simulink model "ACC_Scenario_006_cs"  (R2014b)
settings: Solver=ode5  SolverMode=SingleTasking  StartTime=0.0  StopTime=inf  FixedStep=1/100  RelTol=1e-3
PreLoadFcn:
  | mbxruntime.callbacks.PreLoadFcn(bdroot);
  | check_NUTS_defined;
  | 
  | assignin('base',['model_closed_' bdroot],false);addpath('../includes_ACC');
PostLoadFcn:
  | mbxruntime.callbacks.PostLoadFcn(bdroot);
InitFcn:
  | mbxruntime.callbacks.InitFcn(bdroot);
StartFcn:
  | mbxruntime.callbacks.StartFcn(bdroot);
StopFcn:
  | mbxruntime.callbacks.StopFcn(bdroot);
model workspace: external: MAT-File .\ACC_Scenario_006_cs_hws.mat (data not in the file)
undefined symbols (not defined in the file or in its folder): mbxruntime, OrientationPitch, OrientationRoll, PositionX, PositionY, PositionZ, tabledata, warningInitialVelocity, x0
undefined symbols (not defined in the file): ACC_Scenario_006_cs_061450488d6753c4, ACC_Scenario_006_cs_13896134c615b72a, ACC_Scenario_006_cs_18eaf2a52f2ef75d, ACC_Scenario_006_cs_59e375456829d2f0, ACC_Scenario_006_cs_8a2109b915871f11, ACC_Scenario_006_cs_a4f79cab717c06e2, ACC_Scenario_006_cs_Audi_A8_1_Dynamics_Simple_initialPitch, ACC_Scenario_006_cs_Audi_A8_1_Dynamics_Simple_initialRoll, ACC_Scenario_006_cs_Audi_A8_1_Dynamics_Simple_initialX, ACC_Scenario_006_cs_Audi_A8_1_Dynamics_Simple_initialY, ACC_Scenario_006_cs_Audi_A8_1_Dynamics_Simple_initialYaw, ACC_Scenario_006_cs_Audi_A8_1_Dynamics_Simple_initialZ, ACC_Scenario_006_cs_BMW_X5_1_Path_pathUniqueID, ACC_Scenario_006_cs_BMW_X5_1_SpeedProfile_speedProfileUniqueID, ACC_Scenario_006_cs_e4633c18fd34a832, ACC_Scenario_006_cs_f83c81dc10cd364a, ACC_Scenario_006_cs_Fiat_Bravo_1_Path_pathUniqueID, ACC_Scenario_006_cs_Ford_Fiesta_1_Path_pathUniqueID, ACC_Scenario_006_cs_Honda_Pan_European_1_Path_pathUniqueID, ACC_Scenario_006_cs_Mazda_RX8_1_Path_pathUniqueID, ACC_Scenario_006_cs_Sphere_1_Dynamics_Empty_STATE_Sphere_1_x0, ACC_Scenario_006_cs_Sphere_1_Dynamics_Empty_STATE_Sphere_1_y0, ACC_Scenario_006_cs_Sphere_1_Dynamics_Empty_STATE_Sphere_1_Yaw0, ACC_Scenario_006_cs_Sphere_1_Dynamics_Empty_STATE_Sphere_1_z0, ACC_Scenario_006_cs_Toyota_Yaris_1_Path_pathUniqueID, SteeringColumn, SteeringWheel, Wheel0, Wheel0_Suspension, Wheel1, Wheel1_Suspension, WheelL0, WheelL1, WheelR0, WheelR1
libraries: simulink_extras x60, simulink x21, PreScanSimulinkLibrary x5, PreScanUsefulBlocks x2
(part 9 of 24)

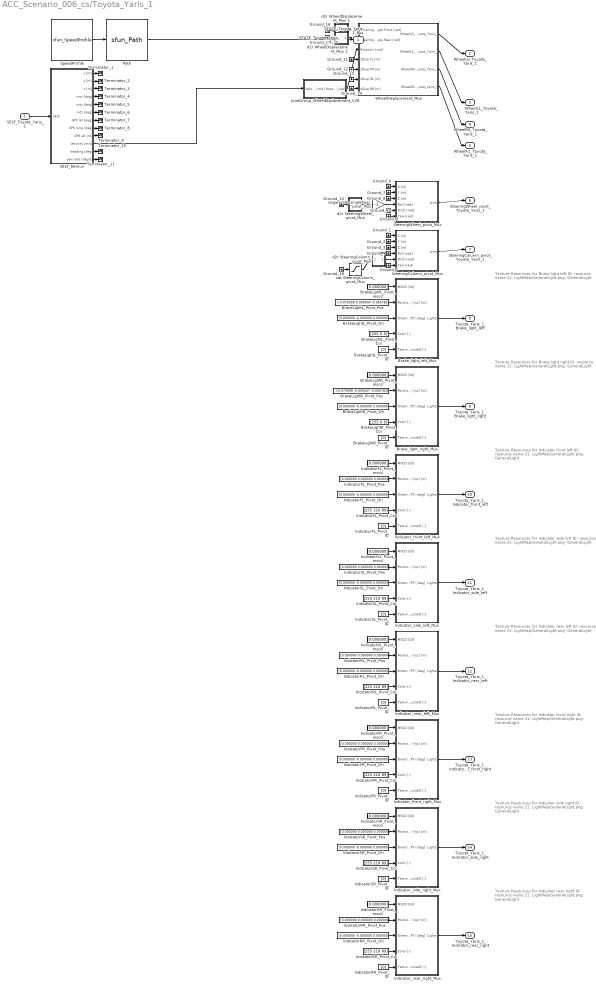
== system ACC_Scenario_006_cs/Toyota_Yaris_1 ==
  note: Texture Resources for Brake light left
      |
      | ID: resource name
      | 21: LightMap\GeneralLight.png: GeneralLight
  note: Texture Resources for Brake light right
      |
      | ID: resource name
      | 21: LightMap\GeneralLight.png: GeneralLight
  note: Texture Resources for Indicator front left
      |
      | ID: resource name
      | 21: LightMap\GeneralLight.png: GeneralLight
  note: Texture Resources for Indicator side left
      |
      | ID: resource name
      | 21: LightMap\GeneralLight.png: GeneralLight
  note: Texture Resources for Indicator rear left
      |
      | ID: resource name
      | 21: LightMap\GeneralLight.png: GeneralLight
  note: Texture Resources for Indicator front right
      |
      | ID: resource name
      | 21: LightMap\GeneralLight.png: GeneralLight
  note: Texture Resources for Indicator side right
      |
      | ID: resource name
      | 21: LightMap\GeneralLight.png: GeneralLight
  note: Texture Resources for Indicator rear right
      |
      | ID: resource name
      | 21: LightMap\GeneralLight.png: GeneralLight
  SELF_Toyota_Yaris_1 : Inport  Tag=inport/SelfPort  OutDataTypeStr=Bus: PRESCAN_SELFSENSORDATA  PortDimensions=1  SampleTime=1/100  BusOutputAsStruct=on
  BrakeLightL_Pivot_Col : Constant  Tag=VisuLightConst  Value=[255 0 0]
  BrakeLightL_Pivot_ID : Constant  Tag=VisuLightConst  Value=[0]
  BrakeLightL_Pivot_Ori : Constant  Tag=VisuLightConst  Value=[0.000000 -0.000000 0.000000]
  BrakeLightL_Pivot_Pos : Constant  Tag=VisuLightConst  Value=[-0.073098 0.009000 -0.060782]
  BrakeLightL_Pivot_mscd : Constant  Tag=VisuLightConst  Value=[0.000000]
  BrakeLightR_Pivot_Col : Constant  Tag=VisuLightConst  Value=[255 0 0]
  BrakeLightR_Pivot_ID : Constant  Tag=VisuLightConst  Value=[0]
  BrakeLightR_Pivot_Ori : Constant  Tag=VisuLightConst  Value=[0.000000 -0.000000 0.000000]
  BrakeLightR_Pivot_Pos : Constant  Tag=VisuLightConst  Value=[-0.073098 -0.009447 -0.060782]
  BrakeLightR_Pivot_mscd : Constant  Tag=VisuLightConst  Value=[0.000000]
  Brake_light_left_Mux : Subsystem  Tag=mux/ActiveLight  mask(PreScan User Interface: VisuActiveLight){}
      mask help:
      | The VisuActiveLight block provides a way for detailed animation of Light Sources, such as the indicator, brake, fog and main lights of a vehicle, or a light post.
      |
      | For more information, please click Help.
      settings: DeleteFcn=PreScanBlockDeleteFcn;
      mask Help: eval('openHelp(209)')
  Brake_light_right_Mux : Subsystem  Tag=mux/ActiveLight  mask(PreScan User Interface: VisuActiveLight){}
      mask help:
      | The VisuActiveLight block provides a way for detailed animation of Light Sources, such as the indicator, brake, fog and main lights of a vehicle, or a light post.
      |
      | For more information, please click Help.
      settings: DeleteFcn=PreScanBlockDeleteFcn;
      mask Help: eval('openHelp(209)')
  Ground_{1..18} (18 alike) : Ground
  IndicatorFL_Pivot_Col : Constant  Tag=VisuLightConst  Value=[255 210 89]
  IndicatorFL_Pivot_ID : Constant  Tag=VisuLightConst  Value=[0]
  IndicatorFL_Pivot_Ori : Constant  Tag=VisuLightConst  Value=[0.000000 -0.000000 0.000000]
  IndicatorFL_Pivot_Pos : Constant  Tag=VisuLightConst  Value=[0.000000 0.000000 0.000000]
  IndicatorFL_Pivot_mscd : Constant  Tag=VisuLightConst  Value=[0.000000]
  IndicatorFR_Pivot_Col : Constant  Tag=VisuLightConst  Value=[255 210 89]
  IndicatorFR_Pivot_ID : Constant  Tag=VisuLightConst  Value=[0]
  IndicatorFR_Pivot_Ori : Constant  Tag=VisuLightConst  Value=[0.000000 -0.000000 0.000000]
  IndicatorFR_Pivot_Pos : Constant  Tag=VisuLightConst  Value=[0.000000 0.000000 0.000000]
  IndicatorFR_Pivot_mscd : Constant  Tag=VisuLightConst  Value=[0.000000]
  IndicatorRL_Pivot_Col : Constant  Tag=VisuLightConst  Value=[255 210 89]
  IndicatorRL_Pivot_ID : Constant  Tag=VisuLightConst  Value=[0]
  IndicatorRL_Pivot_Ori : Constant  Tag=VisuLightConst  Value=[0.000000 -0.000000 0.000000]
  IndicatorRL_Pivot_Pos : Constant  Tag=VisuLightConst  Value=[0.000000 0.000000 0.000000]
  IndicatorRL_Pivot_mscd : Constant  Tag=VisuLightConst  Value=[0.000000]
  IndicatorRR_Pivot_Col : Constant  Tag=VisuLightConst  Value=[255 210 89]
  IndicatorRR_Pivot_ID : Constant  Tag=VisuLightConst  Value=[0]
  IndicatorRR_Pivot_Ori : Constant  Tag=VisuLightConst  Value=[0.000000 -0.000000 0.000000]
  IndicatorRR_Pivot_Pos : Constant  Tag=VisuLightConst  Value=[0.000000 0.000000 0.000000]
  IndicatorRR_Pivot_mscd : Constant  Tag=VisuLightConst  Value=[0.000000]
  IndicatorSL_Pivot_Col : Constant  Tag=VisuLightConst  Value=[255 210 89]
  IndicatorSL_Pivot_ID : Constant  Tag=VisuLightConst  Value=[0]
  IndicatorSL_Pivot_Ori : Constant  Tag=VisuLightConst  Value=[0.000000 -0.000000 0.000000]
  IndicatorSL_Pivot_Pos : Constant  Tag=VisuLightConst  Value=[0.000000 0.000000 0.000000]
  IndicatorSL_Pivot_mscd : Constant  Tag=VisuLightConst  Value=[0.000000]
  IndicatorSR_Pivot_Col : Constant  Tag=VisuLightConst  Value=[255 210 89]
  IndicatorSR_Pivot_ID : Constant  Tag=VisuLightConst  Value=[0]
  IndicatorSR_Pivot_Ori : Constant  Tag=VisuLightConst  Value=[0.000000 -0.000000 0.000000]
  IndicatorSR_Pivot_Pos : Constant  Tag=VisuLightConst  Value=[0.000000 0.000000 0.000000]
  IndicatorSR_Pivot_mscd : Constant  Tag=VisuLightConst  Value=[0.000000]
  Indicator_front_left_Mux : Subsystem  Tag=mux/ActiveLight  mask(PreScan User Interface: VisuActiveLight){}
      mask help:
      | The VisuActiveLight block provides a way for detailed animation of Light Sources, such as the indicator, brake, fog and main lights of a vehicle, or a light post.
      |
      | For more information, please click Help.
      settings: DeleteFcn=PreScanBlockDeleteFcn;
      mask Help: eval('openHelp(209)')
  Indicator_front_right_Mux : Subsystem  Tag=mux/ActiveLight  mask(PreScan User Interface: VisuActiveLight){}
      mask help:
      | The VisuActiveLight block provides a way for detailed animation of Light Sources, such as the indicator, brake, fog and main lights of a vehicle, or a light post.
      |
      | For more information, please click Help.
      settings: DeleteFcn=PreScanBlockDeleteFcn;
      mask Help: eval('openHelp(209)')
  Indicator_rear_left_Mux : Subsystem  Tag=mux/ActiveLight  mask(PreScan User Interface: VisuActiveLight){}
      mask help:
      | The VisuActiveLight block provides a way for detailed animation of Light Sources, such as the indicator, brake, fog and main lights of a vehicle, or a light post.
      |
      | For more information, please click Help.
      settings: DeleteFcn=PreScanBlockDeleteFcn;
      mask Help: eval('openHelp(209)')
  Indicator_rear_right_Mux : Subsystem  Tag=mux/ActiveLight  mask(PreScan User Interface: VisuActiveLight){}
      mask help:
      | The VisuActiveLight block provides a way for detailed animation of Light Sources, such as the indicator, brake, fog and main lights of a vehicle, or a light post.
      |
      | For more information, please click Help.
      settings: DeleteFcn=PreScanBlockDeleteFcn;
      mask Help: eval('openHelp(209)')
  Indicator_side_left_Mux : Subsystem  Tag=mux/ActiveLight  mask(PreScan User Interface: VisuActiveLight){}
      mask help:
      | The VisuActiveLight block provides a way for detailed animation of Light Sources, such as the indicator, brake, fog and main lights of a vehicle, or a light post.
      |
      | For more information, please click Help.
      settings: DeleteFcn=PreScanBlockDeleteFcn;
      mask Help: eval('openHelp(209)')
  Indicator_side_right_Mux : Subsystem  Tag=mux/ActiveLight  mask(PreScan User Interface: VisuActiveLight){}
      mask help:
      | The VisuActiveLight block provides a way for detailed animation of Light Sources, such as the indicator, brake, fog and main lights of a vehicle, or a light post.
      |
      | For more information, please click Help.
      settings: DeleteFcn=PreScanBlockDeleteFcn;
      mask Help: eval('openHelp(209)')
  JointGroup_WheelDisplacement_V2R : Subsystem  Tag=mux/Wheels  mask(PreScan Velocity to Wheel Angle Block:){TimeStep=1/100, TireRadius=0.29}
      mask prompts: TimeStep "Auto Assigned: Time Step [s]"; TireRadius "Tire Radius [m]"
      settings: DeleteFcn=PreScanBlockDeleteFcn;
      mask Display: disp('Velocity\nto\nWheelAngle')
  Path : S-Function  Tag=Path  LoadFcn=load('PrescanMotionData.mat')  FunctionName=sfun_Path  Parameters=uniqueID, pathUniqueID, timestep  EnableBusSupport=off  mask(Path){uniqueID=359, pathUniqueID=ACC_Scenario_006_cs_Toyota_Yaris_1_Path_pathUniqueID, timestep=1/100}
      mask prompts: uniqueID "Object Unique ID"; pathUniqueID "Path Unique ID"; timestep "MATLAB timestep:"
      mask help:
      | The path block outputs the position along a given trajectory.
      |
      | For more information, please click Help.
      mask Help: eval('openHelp(312)')
      mask Display: image(imread('Path.png'))
  SELF_Demux : Subsystem  Tag=demux/SelfPort  mask(PreScan Demux Block:){}
      mask help:
      | The SELF port shows (state) information of the actor itself. The outputs are position in the experiment's axis system and the GPS coordinates, and the object's absolute velocity and compass heading.
      |
      | For more information, please click Help.
      settings: DeleteFcn=PreScanBlockDeleteFcn;
      mask Help: eval('openHelp(462)')
      mask Display:
      | port_label('output',1,'x [m]')
      | port_label('output',2,'y [m]')
      | port_label('output',3,'z [m]','texmode','on')
      | port_label('output',4,'Rotx [deg]','texmode','on')
      | port_label('output',5,'Roty [deg]','texmode','on')
      | port_label('output',6,'Rotz [deg]','texmode','on')
      | port_label('output',7,'GPS lat [deg]','texmode','on')
      | port_label('output',8,'GPS long [deg]','texmode','on')
      | port_label('output',9,'GPS alt [m]','texmode','on')
      | port_label('output',10,'Velocity [m/s]')
      | port_label('output',11,'Heading [deg]')
      | port_label('output',12,'Yaw rate [deg/s]')
  STATE_Toyota_Yaris_1_rc : RateTransition  Tag=mux_rc/StatePort  OutPortSampleTimeOpt=Inherit
  SpeedProfile : S-Function  Tag=SpeedProfile  LoadFcn=load('PrescanMotionData.mat')  FunctionName=sfun_SpeedProfile  Parameters=speedProfileUniqueID, timestep  EnableBusSupport=off  mask(SpeedProfile){speedProfileUniqueID=ACC_Scenario_006_cs_13896134c615b72a, timestep=1/100}
      mask prompts: speedProfileUniqueID "Speed Profile Unique ID"; timestep "MATLAB timestep:"
      mask help:
      | The speed profile block outputs the travelled distance, velocities and acceleration along a given path.
      |
      | For more information, please click Help.
      mask Help: eval('openHelp(312)')
      mask Display: image(imread('SpeedProfile.png'))
  SteeringColumn_pivot_Mux : Subsystem  Tag=mux/Joint  mask(PreScan Mux Block){DisplayName=SteeringColumn}
      mask prompts: DisplayName "Display Name"
      mask help:
      | This block simulates a generic joint used for generic models. This joint can be enabled/disabled from the GUI.
      |
      | For more information, please click Help.
      settings: DeleteFcn=PreScanBlockDeleteFcn;
      mask Help: eval('openHelp(254)')
  SteeringWheel_pivot_Mux : Subsystem  Tag=mux/Joint  mask(PreScan Mux Block){DisplayName=SteeringWheel}
      mask prompts: DisplayName "Display Name"
      mask help:
      | This block simulates a generic joint used for generic models. This joint can be enabled/disabled from the GUI.
      |
      | For more information, please click Help.
      settings: DeleteFcn=PreScanBlockDeleteFcn;
      mask Help: eval('openHelp(254)')
  Terminator_{1..11} (11 alike) : Terminator
  WheelDisplacement_Mux : Subsystem  Tag=mux/JointGroup  mask(JointGroup){}
      mask help:
      | The JointGroup allows to control several Joints in one go, as defined for this particular model.
      | For more information, look in the PreScan manual in the section "Model Preparation Tool" -> "Joint Groups"
      |
      | For more information on the Joints simulink interface, press Help.
      mask Help: eval('openHelp(254)')
  d2r SteeringColumn_pivot_Mux : Subsystem  mask(DegreesToRadians){}
      mask help: SimulinkBlocks:simulink_extras:DegreesToRadians_MD
      mask Help: web([docroot '/simulink/ref_extras/degreestoradians.html'])
      mask Display: disp('D2R')
  d2r SteeringWheel_pivot_Mux : Subsystem  mask(DegreesToRadians){}
      mask help: SimulinkBlocks:simulink_extras:DegreesToRadians_MD
      mask Help: web([docroot '/simulink/ref_extras/degreestoradians.html'])
      mask Display: disp('D2R')
  d2r WheelDisplacement_Mux 1 : Subsystem  mask(DegreesToRadians){}
      mask help: SimulinkBlocks:simulink_extras:DegreesToRadians_MD
      mask Help: web([docroot '/simulink/ref_extras/degreestoradians.html'])
      mask Display: disp('D2R')
  d2r WheelDisplacement_Mux 2 : Subsystem  mask(DegreesToRadians){}
      mask help: SimulinkBlocks:simulink_extras:DegreesToRadians_MD
      mask Help: web([docroot '/simulink/ref_extras/degreestoradians.html'])
      mask Display: disp('D2R')
  negate SteeringWheel_pivot_Mux : Gain  Gain=-1
  sat SteeringColumn_pivot_Mux : Saturate  UpperLimit=30  LowerLimit=-5
  STATE_Toyota_Yaris_1_bus : Outport  Tag=outport/StatePort  OutDataTypeStr=Bus: PRESCAN_STATEACTUATORDATA  PortDimensions=1  SampleTime=1/100
  WheelL0_Toyota_Yaris_1 : Outport  Tag=outport/JointActuator  Port=2  OutDataTypeStr=Bus: PRESCAN_POSE_DATA  SampleTime=1/100
  WheelL1_Toyota_Yaris_1 : Outport  Tag=outport/JointActuator  Port=3  OutDataTypeStr=Bus: PRESCAN_POSE_DATA  SampleTime=1/100
  WheelR0_Toyota_Yaris_1 : Outport  Tag=outport/JointActuator  Port=4  OutDataTypeStr=Bus: PRESCAN_POSE_DATA  SampleTime=1/100
  WheelR1_Toyota_Yaris_1 : Outport  Tag=outport/JointActuator  Port=5  OutDataTypeStr=Bus: PRESCAN_POSE_DATA  SampleTime=1/100
  SteeringWheel_pivot_Toyota_Yaris_1 : Outport  Tag=outport/JointActuator  Port=6  OutDataTypeStr=Bus: PRESCAN_POSE_DATA  SampleTime=1/100
  SteeringColumn_pivot_Toyota_Yaris_1 : Outport  Tag=outport/JointActuator  Port=7  OutDataTypeStr=Bus: PRESCAN_POSE_DATA  SampleTime=1/100
  Toyota_Yaris_1_Brake_light_left : Outport  Tag=outport/BrakeLightL_Pivot  Port=8  OutDataTypeStr=Bus: PRESCAN_VISULIGHTACTUATOR_DATA  SampleTime=1/100
  Toyota_Yaris_1_Brake_light_right : Outport  Tag=outport/BrakeLightR_Pivot  Port=9  OutDataTypeStr=Bus: PRESCAN_VISULIGHTACTUATOR_DATA  SampleTime=1/100
  Toyota_Yaris_1_Indicator_front_left : Outport  Tag=outport/IndicatorFL_Pivot  Port=10  OutDataTypeStr=Bus: PRESCAN_VISULIGHTACTUATOR_DATA  SampleTime=1/100
  Toyota_Yaris_1_Indicator_side_left : Outport  Tag=outport/IndicatorSL_Pivot  Port=11  OutDataTypeStr=Bus: PRESCAN_VISULIGHTACTUATOR_DATA  SampleTime=1/100
  Toyota_Yaris_1_Indicator_rear_left : Outport  Tag=outport/IndicatorRL_Pivot  Port=12  OutDataTypeStr=Bus: PRESCAN_VISULIGHTACTUATOR_DATA  SampleTime=1/100
  Toyota_Yaris_1_Indicator_front_right : Outport  Tag=outport/IndicatorFR_Pivot  Port=13  OutDataTypeStr=Bus: PRESCAN_VISULIGHTACTUATOR_DATA  SampleTime=1/100
  Toyota_Yaris_1_Indicator_side_right : Outport  Tag=outport/IndicatorSR_Pivot  Port=14  OutDataTypeStr=Bus: PRESCAN_VISULIGHTACTUATOR_DATA  SampleTime=1/100
  Toyota_Yaris_1_Indicator_rear_right : Outport  Tag=outport/IndicatorRR_Pivot  Port=15  OutDataTypeStr=Bus: PRESCAN_VISULIGHTACTUATOR_DATA  SampleTime=1/100
  wires:
  sat SteeringColumn_pivot_Mux/1 -> d2r SteeringColumn_pivot_Mux/1(Degrees in)
  d2r SteeringColumn_pivot_Mux/1(Radians out) -> SteeringColumn_pivot_Mux/5(Pitch [rad])
  d2r SteeringWheel_pivot_Mux/1(Radians out) -> negate SteeringWheel_pivot_Mux/1
  negate SteeringWheel_pivot_Mux/1 -> SteeringWheel_pivot_Mux/4(Roll [rad])
  d2r WheelDisplacement_Mux 1/1(Radians out) -> WheelDisplacement_Mux/1(Steering Angle Front [rad])
  d2r WheelDisplacement_Mux 2/1(Radians out) -> WheelDisplacement_Mux/2(Steering Angle Rear [rad])
  SELF_Demux/10(velocity [m/s]) -> JointGroup_WheelDisplacement_V2R/1(Velocity [m/s])
  STATE_Toyota_Yaris_1_rc/1 -> STATE_Toyota_Yaris_1_bus/1
  SpeedProfile/1 -> Path/1
  Path/1 -> STATE_Toyota_Yaris_1_rc/1
  SELF_Toyota_Yaris_1/1 -> SELF_Demux/1(SELF)
  WheelDisplacement_Mux/1(WheelL0_Toyota_Yaris_1) -> WheelL0_Toyota_Yaris_1/1
  WheelDisplacement_Mux/2(WheelL1_Toyota_Yaris_1) -> WheelL1_Toyota_Yaris_1/1
  WheelDisplacement_Mux/3(WheelR0_Toyota_Yaris_1) -> WheelR0_Toyota_Yaris_1/1
  WheelDisplacement_Mux/4(WheelR1_Toyota_Yaris_1) -> WheelR1_Toyota_Yaris_1/1
  JointGroup_WheelDisplacement_V2R/1(Rotation [rad]) -> WheelDisplacement_Mux/3(Rotation [rad])
  SteeringWheel_pivot_Mux/1(Joint) -> SteeringWheel_pivot_Toyota_Yaris_1/1
  SteeringColumn_pivot_Mux/1(Joint) -> SteeringColumn_pivot_Toyota_Yaris_1/1
  Brake_light_left_Mux/1(Lights) -> Toyota_Yaris_1_Brake_light_left/1
  BrakeLightL_Pivot_mscd/1 -> Brake_light_left_Mux/1(MSCD [Cd])
  BrakeLightL_Pivot_Pos/1 -> Brake_light_left_Mux/2(Position (xyz) [m])
  BrakeLightL_Pivot_Ori/1 -> Brake_light_left_Mux/3(Orientation (RPY) [deg])
  BrakeLightL_Pivot_Col/1 -> Brake_light_left_Mux/4(Color [-])
  BrakeLightL_Pivot_ID/1 -> Brake_light_left_Mux/5(TextureResourceID [-])
  Brake_light_right_Mux/1(Lights) -> Toyota_Yaris_1_Brake_light_right/1
  BrakeLightR_Pivot_mscd/1 -> Brake_light_right_Mux/1(MSCD [Cd])
  BrakeLightR_Pivot_Pos/1 -> Brake_light_right_Mux/2(Position (xyz) [m])
  BrakeLightR_Pivot_Ori/1 -> Brake_light_right_Mux/3(Orientation (RPY) [deg])
  BrakeLightR_Pivot_Col/1 -> Brake_light_right_Mux/4(Color [-])
  BrakeLightR_Pivot_ID/1 -> Brake_light_right_Mux/5(TextureResourceID [-])
  Indicator_front_left_Mux/1(Lights) -> Toyota_Yaris_1_Indicator_front_left/1
  IndicatorFL_Pivot_mscd/1 -> Indicator_front_left_Mux/1(MSCD [Cd])
  IndicatorFL_Pivot_Pos/1 -> Indicator_front_left_Mux/2(Position (xyz) [m])
  IndicatorFL_Pivot_Ori/1 -> Indicator_front_left_Mux/3(Orientation (RPY) [deg])
  IndicatorFL_Pivot_Col/1 -> Indicator_front_left_Mux/4(Color [-])
  IndicatorFL_Pivot_ID/1 -> Indicator_front_left_Mux/5(TextureResourceID [-])
  Indicator_side_left_Mux/1(Lights) -> Toyota_Yaris_1_Indicator_side_left/1
  IndicatorSL_Pivot_mscd/1 -> Indicator_side_left_Mux/1(MSCD [Cd])
  IndicatorSL_Pivot_Pos/1 -> Indicator_side_left_Mux/2(Position (xyz) [m])
  IndicatorSL_Pivot_Ori/1 -> Indicator_side_left_Mux/3(Orientation (RPY) [deg])
  IndicatorSL_Pivot_Col/1 -> Indicator_side_left_Mux/4(Color [-])
  IndicatorSL_Pivot_ID/1 -> Indicator_side_left_Mux/5(TextureResourceID [-])
  Indicator_rear_left_Mux/1(Lights) -> Toyota_Yaris_1_Indicator_rear_left/1
  IndicatorRL_Pivot_mscd/1 -> Indicator_rear_left_Mux/1(MSCD [Cd])
  IndicatorRL_Pivot_Pos/1 -> Indicator_rear_left_Mux/2(Position (xyz) [m])
  IndicatorRL_Pivot_Ori/1 -> Indicator_rear_left_Mux/3(Orientation (RPY) [deg])
  IndicatorRL_Pivot_Col/1 -> Indicator_rear_left_Mux/4(Color [-])
  IndicatorRL_Pivot_ID/1 -> Indicator_rear_left_Mux/5(TextureResourceID [-])
  Indicator_front_right_Mux/1(Lights) -> Toyota_Yaris_1_Indicator_front_right/1
  IndicatorFR_Pivot_mscd/1 -> Indicator_front_right_Mux/1(MSCD [Cd])
  IndicatorFR_Pivot_Pos/1 -> Indicator_front_right_Mux/2(Position (xyz) [m])
  IndicatorFR_Pivot_Ori/1 -> Indicator_front_right_Mux/3(Orientation (RPY) [deg])
  IndicatorFR_Pivot_Col/1 -> Indicator_front_right_Mux/4(Color [-])
  IndicatorFR_Pivot_ID/1 -> Indicator_front_right_Mux/5(TextureResourceID [-])
  Indicator_side_right_Mux/1(Lights) -> Toyota_Yaris_1_Indicator_side_right/1
  IndicatorSR_Pivot_mscd/1 -> Indicator_side_right_Mux/1(MSCD [Cd])
  IndicatorSR_Pivot_Pos/1 -> Indicator_side_right_Mux/2(Position (xyz) [m])
  IndicatorSR_Pivot_Ori/1 -> Indicator_side_right_Mux/3(Orientation (RPY) [deg])
  IndicatorSR_Pivot_Col/1 -> Indicator_side_right_Mux/4(Color [-])
  IndicatorSR_Pivot_ID/1 -> Indicator_side_right_Mux/5(TextureResourceID [-])
  Indicator_rear_right_Mux/1(Lights) -> Toyota_Yaris_1_Indicator_rear_right/1
  IndicatorRR_Pivot_mscd/1 -> Indicator_rear_right_Mux/1(MSCD [Cd])
  IndicatorRR_Pivot_Pos/1 -> Indicator_rear_right_Mux/2(Position (xyz) [m])
  IndicatorRR_Pivot_Ori/1 -> Indicator_rear_right_Mux/3(Orientation (RPY) [deg])
  IndicatorRR_Pivot_Col/1 -> Indicator_rear_right_Mux/4(Color [-])
  IndicatorRR_Pivot_ID/1 -> Indicator_rear_right_Mux/5(TextureResourceID [-])
  SELF_Demux/1(x [m]) -> Terminator_1/1
  SELF_Demux/2(y [m]) -> Terminator_2/1
  SELF_Demux/3(z [m]) -> Terminator_3/1
  SELF_Demux/4(rotx [deg]) -> Terminator_4/1
  SELF_Demux/5(roty [deg]) -> Terminator_5/1
  SELF_Demux/6(rotz [deg]) -> Terminator_6/1
  SELF_Demux/7(GPS lat [deg]) -> Terminator_7/1
  SELF_Demux/8(GPS long [deg]) -> Terminator_8/1
  SELF_Demux/9(GPS alt [m]) -> Terminator_9/1
  SELF_Demux/11(heading [deg]) -> Terminator_10/1
  SELF_Demux/12(yaw rate [deg/s]) -> Terminator_11/1
  Ground_1/1 -> SteeringColumn_pivot_Mux/1(X [m])
  Ground_2/1 -> SteeringColumn_pivot_Mux/2(Y [m])
  Ground_3/1 -> SteeringColumn_pivot_Mux/3(Z [m])
  Ground_4/1 -> SteeringColumn_pivot_Mux/4(Roll [rad])
  Ground_5/1 -> SteeringColumn_pivot_Mux/6(Yaw [rad])
  Ground_6/1 -> SteeringWheel_pivot_Mux/1(X [m])
  Ground_7/1 -> SteeringWheel_pivot_Mux/2(Y [m])
  Ground_8/1 -> SteeringWheel_pivot_Mux/3(Z [m])
  Ground_9/1 -> SteeringWheel_pivot_Mux/5(Pitch [rad])
  Ground_10/1 -> SteeringWheel_pivot_Mux/6(Yaw [rad])
  Ground_11/1 -> WheelDisplacement_Mux/4(zDisp FL [m])
  Ground_12/1 -> WheelDisplacement_Mux/5(zDisp FR [m])
  Ground_13/1 -> WheelDisplacement_Mux/6(zDisp RL [m])
  Ground_14/1 -> WheelDisplacement_Mux/7(zDisp RR [m])
  Ground_15/1 -> d2r SteeringWheel_pivot_Mux/1(Degrees in)
  Ground_16/1 -> d2r WheelDisplacement_Mux 1/1(Degrees in)
  Ground_17/1 -> d2r WheelDisplacement_Mux 2/1(Degrees in)
  Ground_18/1 -> sat SteeringColumn_pivot_Mux/1

== system ACC_Scenario_006_cs/Toyota_Yaris_1_Brake_light_left ==
  Toyota_Yaris_1_Brake_light_left : Inport  Tag=inport/BrakeLightL_Pivot  OutDataTypeStr=Bus: PRESCAN_VISULIGHTACTUATOR_DATA  SampleTime=1/100  BusOutputAsStruct=on
  Actuator : S-Function  FunctionName=sfun_VisuLightActuator  Parameters=mbxruntime.parameters.convert(UniqueID), mbxruntime.parameters.convert(LightName), mbxruntime.parameters.convert(PivotName), mbxruntime.parameters.convert(TextureResources), mbxruntime.parameters.convert(ColorsObjectName), mbxruntime.parameters.convert(MeshOnColor), mbxruntime.parameters.convert(MeshOffColor),tabledata, TimeStep  EnableBusSupport=off  mask(PreScan Sink Block: VisuActiveLight){UniqueID=359, LightName=Toyota_Yaris_1.LightActuator_0_BrakeLightL_ActiveLight, PivotName=Toyota_Yaris_1.BrakeLightL_Pivot, TextureResources={ '21' 'LightMap\GeneralLight.png'}, ColorsObjectName=Toyota_Yaris_1.BrakeLightL, MeshOnColor=[255    0    0  255  255    0    0  255  102  102  102  255  510    0    0  255], MeshOffColor=[255    0    0  255  255    0    0  255  102  102  102  255    0    0    0  255], TimeStep=1/100}
      mask prompts: UniqueID "Parent Unique Identifier"; LightName "Light"; PivotName "Pivot"; TextureResources "Texture Resources"; ColorsObjectName "Light Fixture Color Object"; MeshOnColor "Light Fixture On Color"; MeshOffColor "Light Fixture Off Color"; TimeStep "Simulink time step"
      mask help:
      | The VisuActiveLight block provides a way for detailed animation of Light Sources, such as the indicator, brake, fog and main lights of a vehicle, or a light post.
      |
      | For more information, please click Help.
      mask init:
      | [tabledata] = mbxruntime.parameters.table(UniqueID,LightName,PivotName,TextureResources,ColorsObjectName,MeshOnColor,MeshOffColor);
      mask Help: eval('openHelp(209)')
      mask Display: image(imread('HeadLight.png'))
  wires:
  Toyota_Yaris_1_Brake_light_left/1 -> Actuator/1

== system ACC_Scenario_006_cs/Toyota_Yaris_1_Brake_light_right ==
  Toyota_Yaris_1_Brake_light_right : Inport  Tag=inport/BrakeLightR_Pivot  OutDataTypeStr=Bus: PRESCAN_VISULIGHTACTUATOR_DATA  SampleTime=1/100  BusOutputAsStruct=on
  Actuator : S-Function  FunctionName=sfun_VisuLightActuator  Parameters=mbxruntime.parameters.convert(UniqueID), mbxruntime.parameters.convert(LightName), mbxruntime.parameters.convert(PivotName), mbxruntime.parameters.convert(TextureResources), mbxruntime.parameters.convert(ColorsObjectName), mbxruntime.parameters.convert(MeshOnColor), mbxruntime.parameters.convert(MeshOffColor),tabledata, TimeStep  EnableBusSupport=off  mask(PreScan Sink Block: VisuActiveLight){UniqueID=359, LightName=Toyota_Yaris_1.LightActuator_1_BrakeLightR_ActiveLight, PivotName=Toyota_Yaris_1.BrakeLightR_Pivot, TextureResources={ '21' 'LightMap\GeneralLight.png'}, ColorsObjectName=Toyota_Yaris_1.BrakeLightR, MeshOnColor=[255    0    0  255  255    0    0  255  102  102  102  255  510    0    0  255], MeshOffColor=[255    0    0  255  255    0    0  255  102  102  102  255    0    0    0  255], TimeStep=1/100}
      mask prompts: UniqueID "Parent Unique Identifier"; LightName "Light"; PivotName "Pivot"; TextureResources "Texture Resources"; ColorsObjectName "Light Fixture Color Object"; MeshOnColor "Light Fixture On Color"; MeshOffColor "Light Fixture Off Color"; TimeStep "Simulink time step"
      mask help:
      | The VisuActiveLight block provides a way for detailed animation of Light Sources, such as the indicator, brake, fog and main lights of a vehicle, or a light post.
      |
      | For more information, please click Help.
      mask init:
      | [tabledata] = mbxruntime.parameters.table(UniqueID,LightName,PivotName,TextureResources,ColorsObjectName,MeshOnColor,MeshOffColor);
      mask Help: eval('openHelp(209)')
      mask Display: image(imread('HeadLight.png'))
  wires:
  Toyota_Yaris_1_Brake_light_right/1 -> Actuator/1

== system ACC_Scenario_006_cs/Toyota_Yaris_1_Indicator_front_left ==
  Toyota_Yaris_1_Indicator_front_left : Inport  Tag=inport/IndicatorFL_Pivot  OutDataTypeStr=Bus: PRESCAN_VISULIGHTACTUATOR_DATA  SampleTime=1/100  BusOutputAsStruct=on
  Actuator : S-Function  FunctionName=sfun_VisuLightActuator  Parameters=mbxruntime.parameters.convert(UniqueID), mbxruntime.parameters.convert(LightName), mbxruntime.parameters.convert(PivotName), mbxruntime.parameters.convert(TextureResources), mbxruntime.parameters.convert(ColorsObjectName), mbxruntime.parameters.convert(MeshOnColor), mbxruntime.parameters.convert(MeshOffColor),tabledata, TimeStep  EnableBusSupport=off  mask(PreScan Sink Block: VisuActiveLight){UniqueID=359, LightName=Toyota_Yaris_1.LightActuator_6_IndicatorFL_ActiveLight, PivotName=Toyota_Yaris_1.IndicatorFL_Pivot, TextureResources={ '21' 'LightMap\GeneralLight.png'}, ColorsObjectName=Toyota_Yaris_1.IndicatorFL, MeshOnColor=[255  165    0    0  255  165    0    0  102  102  102  255  510  420  178  255], MeshOffColor=[255  165    0    0  255  165    0    0  102  102  102  255    0    0    0  255], TimeStep=1/100}
      mask prompts: UniqueID "Parent Unique Identifier"; LightName "Light"; PivotName "Pivot"; TextureResources "Texture Resources"; ColorsObjectName "Light Fixture Color Object"; MeshOnColor "Light Fixture On Color"; MeshOffColor "Light Fixture Off Color"; TimeStep "Simulink time step"
      mask help:
      | The VisuActiveLight block provides a way for detailed animation of Light Sources, such as the indicator, brake, fog and main lights of a vehicle, or a light post.
      |
      | For more information, please click Help.
      mask init:
      | [tabledata] = mbxruntime.parameters.table(UniqueID,LightName,PivotName,TextureResources,ColorsObjectName,MeshOnColor,MeshOffColor);
      mask Help: eval('openHelp(209)')
      mask Display: image(imread('HeadLight.png'))
  wires:
  Toyota_Yaris_1_Indicator_front_left/1 -> Actuator/1

== system ACC_Scenario_006_cs/Toyota_Yaris_1_Indicator_front_right ==
  Toyota_Yaris_1_Indicator_front_right : Inport  Tag=inport/IndicatorFR_Pivot  OutDataTypeStr=Bus: PRESCAN_VISULIGHTACTUATOR_DATA  SampleTime=1/100  BusOutputAsStruct=on
  Actuator : S-Function  FunctionName=sfun_VisuLightActuator  Parameters=mbxruntime.parameters.convert(UniqueID), mbxruntime.parameters.convert(LightName), mbxruntime.parameters.convert(PivotName), mbxruntime.parameters.convert(TextureResources), mbxruntime.parameters.convert(ColorsObjectName), mbxruntime.parameters.convert(MeshOnColor), mbxruntime.parameters.convert(MeshOffColor),tabledata, TimeStep  EnableBusSupport=off  mask(PreScan Sink Block: VisuActiveLight){UniqueID=359, LightName=Toyota_Yaris_1.LightActuator_9_IndicatorFR_ActiveLight, PivotName=Toyota_Yaris_1.IndicatorFR_Pivot, TextureResources={ '21' 'LightMap\GeneralLight.png'}, ColorsObjectName=Toyota_Yaris_1.IndicatorFR, MeshOnColor=[255  165    0    0  255  165    0    0  102  102  102  255  510  420  178  255], MeshOffColor=[255  165    0    0  255  165    0    0  102  102  102  255    0    0    0  255], TimeStep=1/100}
      mask prompts: UniqueID "Parent Unique Identifier"; LightName "Light"; PivotName "Pivot"; TextureResources "Texture Resources"; ColorsObjectName "Light Fixture Color Object"; MeshOnColor "Light Fixture On Color"; MeshOffColor "Light Fixture Off Color"; TimeStep "Simulink time step"
      mask help:
      | The VisuActiveLight block provides a way for detailed animation of Light Sources, such as the indicator, brake, fog and main lights of a vehicle, or a light post.
      |
      | For more information, please click Help.
      mask init:
      | [tabledata] = mbxruntime.parameters.table(UniqueID,LightName,PivotName,TextureResources,ColorsObjectName,MeshOnColor,MeshOffColor);
      mask Help: eval('openHelp(209)')
      mask Display: image(imread('HeadLight.png'))
  wires:
  Toyota_Yaris_1_Indicator_front_right/1 -> Actuator/1

== system ACC_Scenario_006_cs/Toyota_Yaris_1_Indicator_rear_left ==
  Toyota_Yaris_1_Indicator_rear_left : Inport  Tag=inport/IndicatorRL_Pivot  OutDataTypeStr=Bus: PRESCAN_VISULIGHTACTUATOR_DATA  SampleTime=1/100  BusOutputAsStruct=on
  Actuator : S-Function  FunctionName=sfun_VisuLightActuator  Parameters=mbxruntime.parameters.convert(UniqueID), mbxruntime.parameters.convert(LightName), mbxruntime.parameters.convert(PivotName), mbxruntime.parameters.convert(TextureResources), mbxruntime.parameters.convert(ColorsObjectName), mbxruntime.parameters.convert(MeshOnColor), mbxruntime.parameters.convert(MeshOffColor),tabledata, TimeStep  EnableBusSupport=off  mask(PreScan Sink Block: VisuActiveLight){UniqueID=359, LightName=Toyota_Yaris_1.LightActuator_8_IndicatorRL_ActiveLight, PivotName=Toyota_Yaris_1.IndicatorRL_Pivot, TextureResources={ '21' 'LightMap\GeneralLight.png'}, ColorsObjectName=Toyota_Yaris_1.IndicatorRL, MeshOnColor=[255  165    0    0  255  165    0    0  102  102  102  255  510  420  178  255], MeshOffColor=[255  165    0    0  255  165    0    0  102  102  102  255    0    0    0  255], TimeStep=1/100}
      mask prompts: UniqueID "Parent Unique Identifier"; LightName "Light"; PivotName "Pivot"; TextureResources "Texture Resources"; ColorsObjectName "Light Fixture Color Object"; MeshOnColor "Light Fixture On Color"; MeshOffColor "Light Fixture Off Color"; TimeStep "Simulink time step"
      mask help:
      | The VisuActiveLight block provides a way for detailed animation of Light Sources, such as the indicator, brake, fog and main lights of a vehicle, or a light post.
      |
      | For more information, please click Help.
      mask init:
      | [tabledata] = mbxruntime.parameters.table(UniqueID,LightName,PivotName,TextureResources,ColorsObjectName,MeshOnColor,MeshOffColor);
      mask Help: eval('openHelp(209)')
      mask Display: image(imread('HeadLight.png'))
  wires:
  Toyota_Yaris_1_Indicator_rear_left/1 -> Actuator/1

== system ACC_Scenario_006_cs/Toyota_Yaris_1_Indicator_rear_right ==
  Toyota_Yaris_1_Indicator_rear_right : Inport  Tag=inport/IndicatorRR_Pivot  OutDataTypeStr=Bus: PRESCAN_VISULIGHTACTUATOR_DATA  SampleTime=1/100  BusOutputAsStruct=on
  Actuator : S-Function  FunctionName=sfun_VisuLightActuator  Parameters=mbxruntime.parameters.convert(UniqueID), mbxruntime.parameters.convert(LightName), mbxruntime.parameters.convert(PivotName), mbxruntime.parameters.convert(TextureResources), mbxruntime.parameters.convert(ColorsObjectName), mbxruntime.parameters.convert(MeshOnColor), mbxruntime.parameters.convert(MeshOffColor),tabledata, TimeStep  EnableBusSupport=off  mask(PreScan Sink Block: VisuActiveLight){UniqueID=359, LightName=Toyota_Yaris_1.LightActuator_11_IndicatorRR_ActiveLight, PivotName=Toyota_Yaris_1.IndicatorRR_Pivot, TextureResources={ '21' 'LightMap\GeneralLight.png'}, ColorsObjectName=Toyota_Yaris_1.IndicatorRR, MeshOnColor=[255  165    0    0  255  165    0    0  102  102  102  255  510  420  178  255], MeshOffColor=[255  165    0    0  255  165    0    0  102  102  102  255    0    0    0  255], TimeStep=1/100}
      mask prompts: UniqueID "Parent Unique Identifier"; LightName "Light"; PivotName "Pivot"; TextureResources "Texture Resources"; ColorsObjectName "Light Fixture Color Object"; MeshOnColor "Light Fixture On Color"; MeshOffColor "Light Fixture Off Color"; TimeStep "Simulink time step"
      mask help:
      | The VisuActiveLight block provides a way for detailed animation of Light Sources, such as the indicator, brake, fog and main lights of a vehicle, or a light post.
      |
      | For more information, please click Help.
      mask init:
      | [tabledata] = mbxruntime.parameters.table(UniqueID,LightName,PivotName,TextureResources,ColorsObjectName,MeshOnColor,MeshOffColor);
      mask Help: eval('openHelp(209)')
      mask Display: image(imread('HeadLight.png'))
  wires:
  Toyota_Yaris_1_Indicator_rear_right/1 -> Actuator/1

== system ACC_Scenario_006_cs/Toyota_Yaris_1_Indicator_side_left ==
  Toyota_Yaris_1_Indicator_side_left : Inport  Tag=inport/IndicatorSL_Pivot  OutDataTypeStr=Bus: PRESCAN_VISULIGHTACTUATOR_DATA  SampleTime=1/100  BusOutputAsStruct=on
  Actuator : S-Function  FunctionName=sfun_VisuLightActuator  Parameters=mbxruntime.parameters.convert(UniqueID), mbxruntime.parameters.convert(LightName), mbxruntime.parameters.convert(PivotName), mbxruntime.parameters.convert(TextureResources), mbxruntime.parameters.convert(ColorsObjectName), mbxruntime.parameters.convert(MeshOnColor), mbxruntime.parameters.convert(MeshOffColor),tabledata, TimeStep  EnableBusSupport=off  mask(PreScan Sink Block: VisuActiveLight){UniqueID=359, LightName=Toyota_Yaris_1.LightActuator_7_IndicatorSL_ActiveLight, PivotName=Toyota_Yaris_1.IndicatorSL_Pivot, TextureResources={ '21' 'LightMap\GeneralLight.png'}, ColorsObjectName=Toyota_Yaris_1.IndicatorSL, MeshOnColor=[255  165    0    0  255  165    0    0  102  102  102  255  510  420  178  255], MeshOffColor=[255  165    0    0  255  165    0    0  102  102  102  255    0    0    0  255], TimeStep=1/100}
      mask prompts: UniqueID "Parent Unique Identifier"; LightName "Light"; PivotName "Pivot"; TextureResources "Texture Resources"; ColorsObjectName "Light Fixture Color Object"; MeshOnColor "Light Fixture On Color"; MeshOffColor "Light Fixture Off Color"; TimeStep "Simulink time step"
      mask help:
      | The VisuActiveLight block provides a way for detailed animation of Light Sources, such as the indicator, brake, fog and main lights of a vehicle, or a light post.
      |
      | For more information, please click Help.
      mask init:
      | [tabledata] = mbxruntime.parameters.table(UniqueID,LightName,PivotName,TextureResources,ColorsObjectName,MeshOnColor,MeshOffColor);
      mask Help: eval('openHelp(209)')
      mask Display: image(imread('HeadLight.png'))
  wires:
  Toyota_Yaris_1_Indicator_side_left/1 -> Actuator/1

== system ACC_Scenario_006_cs/Toyota_Yaris_1_Indicator_side_right ==
  Toyota_Yaris_1_Indicator_side_right : Inport  Tag=inport/IndicatorSR_Pivot  OutDataTypeStr=Bus: PRESCAN_VISULIGHTACTUATOR_DATA  SampleTime=1/100  BusOutputAsStruct=on
  Actuator : S-Function  FunctionName=sfun_VisuLightActuator  Parameters=mbxruntime.parameters.convert(UniqueID), mbxruntime.parameters.convert(LightName), mbxruntime.parameters.convert(PivotName), mbxruntime.parameters.convert(TextureResources), mbxruntime.parameters.convert(ColorsObjectName), mbxruntime.parameters.convert(MeshOnColor), mbxruntime.parameters.convert(MeshOffColor),tabledata, TimeStep  EnableBusSupport=off  mask(PreScan Sink Block: VisuActiveLight){UniqueID=359, LightName=Toyota_Yaris_1.LightActuator_10_IndicatorSR_ActiveLight, PivotName=Toyota_Yaris_1.IndicatorSR_Pivot, TextureResources={ '21' 'LightMap\GeneralLight.png'}, ColorsObjectName=Toyota_Yaris_1.IndicatorSR, MeshOnColor=[255  165    0    0  255  165    0    0  102  102  102  255  510  420  178  255], MeshOffColor=[255  165    0    0  255  165    0    0  102  102  102  255    0    0    0  255], TimeStep=1/100}
      mask prompts: UniqueID "Parent Unique Identifier"; LightName "Light"; PivotName "Pivot"; TextureResources "Texture Resources"; ColorsObjectName "Light Fixture Color Object"; MeshOnColor "Light Fixture On Color"; MeshOffColor "Light Fixture Off Color"; TimeStep "Simulink time step"
      mask help:
      | The VisuActiveLight block provides a way for detailed animation of Light Sources, such as the indicator, brake, fog and main lights of a vehicle, or a light post.
      |
      | For more information, please click Help.
      mask init:
      | [tabledata] = mbxruntime.parameters.table(UniqueID,LightName,PivotName,TextureResources,ColorsObjectName,MeshOnColor,MeshOffColor);
      mask Help: eval('openHelp(209)')
      mask Display: image(imread('HeadLight.png'))
  wires:
  Toyota_Yaris_1_Indicator_side_right/1 -> Actuator/1

== system ACC_Scenario_006_cs/VISUMatrixSignLights_HighwayOverhang_1 ==
  VISUMatrixSignLights_HighwayOverhang_1 : Inport  Tag=inport/VisuMatrixSignLights  SampleTime=1/100  BusOutputAsStruct=on
  Actuator : Subsystem  mask(PreScan Sink Block: VisuMatrixSignLights){UniqueID=109, ColorsObjectQuery=, Colors=[]}
      mask prompts: UniqueID "Parent Unique Identifier"; ColorsObjectQuery "Query for Color Object"; Colors "Matrix of colors"
      mask help:
      | The VisuMatrixSignLights block provides a way to switch the lights on the matrix sign board on or off
      |
      | For more information, please click Help.
      mask Help: eval('openHelp(732)')
      mask Display: image(imread('RearLight.png'))
  wires:
  VISUMatrixSignLights_HighwayOverhang_1/1 -> Actuator/1(VISUMatrixSignLights_HighwayOverhang_1)

== system ACC_Scenario_006_cs/VISUMatrixSignLights_HighwayOverhang_11 ==
  VISUMatrixSignLights_HighwayOverhang_11 : Inport  Tag=inport/VisuMatrixSignLights  SampleTime=1/100  BusOutputAsStruct=on
  Actuator : Subsystem  mask(PreScan Sink Block: VisuMatrixSignLights){UniqueID=120, ColorsObjectQuery=, Colors=[]}
      mask prompts: UniqueID "Parent Unique Identifier"; ColorsObjectQuery "Query for Color Object"; Colors "Matrix of colors"
      mask help:
      | The VisuMatrixSignLights block provides a way to switch the lights on the matrix sign board on or off
      |
      | For more information, please click Help.
      mask Help: eval('openHelp(732)')
      mask Display: image(imread('RearLight.png'))
  wires:
  VISUMatrixSignLights_HighwayOverhang_11/1 -> Actuator/1(VISUMatrixSignLights_HighwayOverhang_11)

== system ACC_Scenario_006_cs/VISUMatrixSignLights_HighwayOverhang_12 ==
  VISUMatrixSignLights_HighwayOverhang_12 : Inport  Tag=inport/VisuMatrixSignLights  SampleTime=1/100  BusOutputAsStruct=on
  Actuator : Subsystem  mask(PreScan Sink Block: VisuMatrixSignLights){UniqueID=121, ColorsObjectQuery=, Colors=[]}
      mask prompts: UniqueID "Parent Unique Identifier"; ColorsObjectQuery "Query for Color Object"; Colors "Matrix of colors"
      mask help:
      | The VisuMatrixSignLights block provides a way to switch the lights on the matrix sign board on or off
      |
      | For more information, please click Help.
      mask Help: eval('openHelp(732)')
      mask Display: image(imread('RearLight.png'))
  wires:
  VISUMatrixSignLights_HighwayOverhang_12/1 -> Actuator/1(VISUMatrixSignLights_HighwayOverhang_12)

== system ACC_Scenario_006_cs/VISUMatrixSignLights_HighwayOverhang_2 ==
  VISUMatrixSignLights_HighwayOverhang_2 : Inport  Tag=inport/VisuMatrixSignLights  SampleTime=1/100  BusOutputAsStruct=on
  Actuator : Subsystem  mask(PreScan Sink Block: VisuMatrixSignLights){UniqueID=110, ColorsObjectQuery=, Colors=[]}
      mask prompts: UniqueID "Parent Unique Identifier"; ColorsObjectQuery "Query for Color Object"; Colors "Matrix of colors"
      mask help:
      | The VisuMatrixSignLights block provides a way to switch the lights on the matrix sign board on or off
      |
      | For more information, please click Help.
      mask Help: eval('openHelp(732)')
      mask Display: image(imread('RearLight.png'))
  wires:
  VISUMatrixSignLights_HighwayOverhang_2/1 -> Actuator/1(VISUMatrixSignLights_HighwayOverhang_2)

== system ACC_Scenario_006_cs/VISUMatrixSign_HighwayOverhang_1 ==
  VISUMatrixSign_HighwayOverhang_1 : Inport  Tag=inport/VisuMatrixSign  SampleTime=1/100  BusOutputAsStruct=on
  Actuator : Subsystem  mask(PreScan Sink Block: VisuMatrixSign){UniqueID=109, ResourceList={'1' 'InformationSign\MatrixSign_GreenArrow.png' '2' 'InformationSign\sign1.jpg' '3' 'InformationSign\sign2.jpg' '4' 'InformationSign\sign3.jpg' '5' 'InformationSign\sign10.png' '7' 'InformationSign\SEARCH_Logo.png' '8' 'InformationSign\sharp_edges.jpg' '9' 'InformationSign\road_surprises.jpg' '10' 'InformationSign\sign5.JPG' '11' 'InformationSign\tacos.jpg' '12' 'InformationSign\dont_even_think.jpg' '13' 'InformationSign\cthulhuwarn.jpg' '14' 'InformationSign\sign7.JPG' '15' 'InformationSign\sign32.jpg' '16' 'InformationSign\NoParking.jpg' '17' 'InformationSign\TheFuture.jpg' '18' 'InformationSign\sign4.jpg' '19' 'InformationSign\sign31.jpg' '20' 'InformationSign\Empty.jpeg' }, PivotName=}
      mask prompts: UniqueID "Parent Unique Identifier (auto-generated)"; ResourceList "Resource List (auto-generated)"; PivotName "Name of pivot (auto-generated)"
      mask help:
      | The VisuMatrixSign block provides a way to adapt the texture of the plates connected to an overhang, based on Resource IDs of the texture files.
      |
      | For more information, please click Help.
      mask Help: eval('openHelp(733)')
      mask Display: image(imread('HighwaySpeedMatrix.png'))
  wires:
  VISUMatrixSign_HighwayOverhang_1/1 -> Actuator/1(VISUMatrixSign_HighwayOverhang_1)

== system ACC_Scenario_006_cs/VISUMatrixSign_HighwayOverhang_10 ==
  VISUMatrixSign_HighwayOverhang_10 : Inport  Tag=inport/VisuMatrixSign  SampleTime=1/100  BusOutputAsStruct=on
  Actuator : Subsystem  mask(PreScan Sink Block: VisuMatrixSign){UniqueID=119, ResourceList={'1' 'InformationSign\MatrixSign_GreenArrow.png' '2' 'InformationSign\sign1.jpg' '3' 'InformationSign\sign2.jpg' '4' 'InformationSign\sign3.jpg' '5' 'InformationSign\sign10.png' '7' 'InformationSign\SEARCH_Logo.png' '8' 'InformationSign\sharp_edges.jpg' '9' 'InformationSign\road_surprises.jpg' '10' 'InformationSign\sign5.JPG' '11' 'InformationSign\tacos.jpg' '12' 'InformationSign\dont_even_think.jpg' '13' 'InformationSign\cthulhuwarn.jpg' '14' 'InformationSign\sign7.JPG' '15' 'InformationSign\sign32.jpg' '16' 'InformationSign\NoParking.jpg' '17' 'InformationSign\TheFuture.jpg' '18' 'InformationSign\sign4.jpg' '19' 'InformationSign\sign31.jpg' '20' 'InformationSign\Empty.jpeg' }, PivotName=}
      mask prompts: UniqueID "Parent Unique Identifier (auto-generated)"; ResourceList "Resource List (auto-generated)"; PivotName "Name of pivot (auto-generated)"
      mask help:
      | The VisuMatrixSign block provides a way to adapt the texture of the plates connected to an overhang, based on Resource IDs of the texture files.
      |
      | For more information, please click Help.
      mask Help: eval('openHelp(733)')
      mask Display: image(imread('HighwaySpeedMatrix.png'))
  wires:
  VISUMatrixSign_HighwayOverhang_10/1 -> Actuator/1(VISUMatrixSign_HighwayOverhang_10)

== system ACC_Scenario_006_cs/VISUMatrixSign_HighwayOverhang_11 ==
  VISUMatrixSign_HighwayOverhang_11 : Inport  Tag=inport/VisuMatrixSign  SampleTime=1/100  BusOutputAsStruct=on
  Actuator : Subsystem  mask(PreScan Sink Block: VisuMatrixSign){UniqueID=120, ResourceList={'1' 'InformationSign\MatrixSign_GreenArrow.png' '2' 'InformationSign\sign1.jpg' '3' 'InformationSign\sign2.jpg' '4' 'InformationSign\sign3.jpg' '5' 'InformationSign\sign10.png' '7' 'InformationSign\SEARCH_Logo.png' '8' 'InformationSign\sharp_edges.jpg' '9' 'InformationSign\road_surprises.jpg' '10' 'InformationSign\sign5.JPG' '11' 'InformationSign\tacos.jpg' '12' 'InformationSign\dont_even_think.jpg' '13' 'InformationSign\cthulhuwarn.jpg' '14' 'InformationSign\sign7.JPG' '15' 'InformationSign\sign32.jpg' '16' 'InformationSign\NoParking.jpg' '17' 'InformationSign\TheFuture.jpg' '18' 'InformationSign\sign4.jpg' '19' 'InformationSign\sign31.jpg' '20' 'InformationSign\Empty.jpeg' }, PivotName=}
      mask prompts: UniqueID "Parent Unique Identifier (auto-generated)"; ResourceList "Resource List (auto-generated)"; PivotName "Name of pivot (auto-generated)"
      mask help:
      | The VisuMatrixSign block provides a way to adapt the texture of the plates connected to an overhang, based on Resource IDs of the texture files.
      |
      | For more information, please click Help.
      mask Help: eval('openHelp(733)')
      mask Display: image(imread('HighwaySpeedMatrix.png'))
  wires:
  VISUMatrixSign_HighwayOverhang_11/1 -> Actuator/1(VISUMatrixSign_HighwayOverhang_11)

== system ACC_Scenario_006_cs/VISUMatrixSign_HighwayOverhang_12 ==
  VISUMatrixSign_HighwayOverhang_12 : Inport  Tag=inport/VisuMatrixSign  SampleTime=1/100  BusOutputAsStruct=on
  Actuator : Subsystem  mask(PreScan Sink Block: VisuMatrixSign){UniqueID=121, ResourceList={'1' 'InformationSign\MatrixSign_GreenArrow.png' '2' 'InformationSign\sign1.jpg' '3' 'InformationSign\sign2.jpg' '4' 'InformationSign\sign3.jpg' '5' 'InformationSign\sign10.png' '7' 'InformationSign\SEARCH_Logo.png' '8' 'InformationSign\sharp_edges.jpg' '9' 'InformationSign\road_surprises.jpg' '10' 'InformationSign\sign5.JPG' '11' 'InformationSign\tacos.jpg' '12' 'InformationSign\dont_even_think.jpg' '13' 'InformationSign\cthulhuwarn.jpg' '14' 'InformationSign\sign7.JPG' '15' 'InformationSign\sign32.jpg' '16' 'InformationSign\NoParking.jpg' '17' 'InformationSign\TheFuture.jpg' '18' 'InformationSign\sign4.jpg' '19' 'InformationSign\sign31.jpg' '20' 'InformationSign\Empty.jpeg' }, PivotName=}
      mask prompts: UniqueID "Parent Unique Identifier (auto-generated)"; ResourceList "Resource List (auto-generated)"; PivotName "Name of pivot (auto-generated)"
      mask help:
      | The VisuMatrixSign block provides a way to adapt the texture of the plates connected to an overhang, based on Resource IDs of the texture files.
      |
      | For more information, please click Help.
      mask Help: eval('openHelp(733)')
      mask Display: image(imread('HighwaySpeedMatrix.png'))
  wires:
  VISUMatrixSign_HighwayOverhang_12/1 -> Actuator/1(VISUMatrixSign_HighwayOverhang_12)

== system ACC_Scenario_006_cs/VISUMatrixSign_HighwayOverhang_2 ==
  VISUMatrixSign_HighwayOverhang_2 : Inport  Tag=inport/VisuMatrixSign  SampleTime=1/100  BusOutputAsStruct=on
  Actuator : Subsystem  mask(PreScan Sink Block: VisuMatrixSign){UniqueID=110, ResourceList={'1' 'InformationSign\MatrixSign_GreenArrow.png' '2' 'InformationSign\sign1.jpg' '3' 'InformationSign\sign2.jpg' '4' 'InformationSign\sign3.jpg' '5' 'InformationSign\sign10.png' '7' 'InformationSign\SEARCH_Logo.png' '8' 'InformationSign\sharp_edges.jpg' '9' 'InformationSign\road_surprises.jpg' '10' 'InformationSign\sign5.JPG' '11' 'InformationSign\tacos.jpg' '12' 'InformationSign\dont_even_think.jpg' '13' 'InformationSign\cthulhuwarn.jpg' '14' 'InformationSign\sign7.JPG' '15' 'InformationSign\sign32.jpg' '16' 'InformationSign\NoParking.jpg' '17' 'InformationSign\TheFuture.jpg' '18' 'InformationSign\sign4.jpg' '19' 'InformationSign\sign31.jpg' '20' 'InformationSign\Empty.jpeg' }, PivotName=}
      mask prompts: UniqueID "Parent Unique Identifier (auto-generated)"; ResourceList "Resource List (auto-generated)"; PivotName "Name of pivot (auto-generated)"
      mask help:
      | The VisuMatrixSign block provides a way to adapt the texture of the plates connected to an overhang, based on Resource IDs of the texture files.
      |
      | For more information, please click Help.
      mask Help: eval('openHelp(733)')
      mask Display: image(imread('HighwaySpeedMatrix.png'))
  wires:
  VISUMatrixSign_HighwayOverhang_2/1 -> Actuator/1(VISUMatrixSign_HighwayOverhang_2)
